simulink model "ModelForAdapt2019"  (R2019b)
settings: Solver=VariableStepAuto  StartTime=0.0  StopTime=i*dt  RelTol=1e-3
values from neighbouring files (symbols this model uses):
  t_sample_est = 0.1    [Filters.m]
undefined symbols (not defined in the file or in its folder): A, B, C, d, E, n_paramConverge, t_observer, x0
libraries: cstblocks x11
settings Model: OrderedModelArguments=off  Creator=micha  LastModifiedBy=gscul
settings DataIOCC: ExternalInput=[u, Ta, Psi]  FinalStateName=OperPoint  InitialState=OperPoint  LoadInitialState=on  SaveFinalState=on  SaveOperatingPoint=on  SaveFormat=StructureWithTime

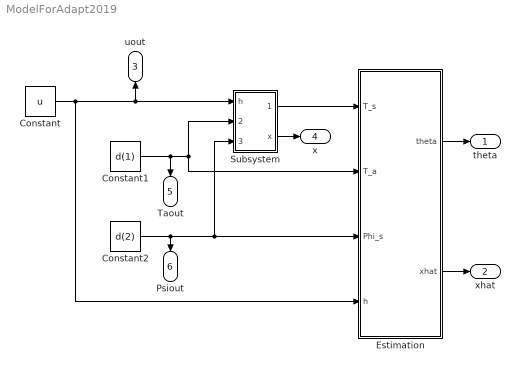
== system ModelForAdapt2019 ==
  Constant : Constant  Value=u
  Constant1 : Constant  Value=d(1)
  Constant2 : Constant  Value=d(2)
  Estimation : Subsystem
  Subsystem : Subsystem
  theta : Outport
  xhat : Outport  Port=2
  uout : Outport  Port=3
  x : Outport  Port=4
  Taout : Outport  Port=5
  Psiout : Outport  Port=6
  wires:
  Subsystem/1(T_s) -> Estimation/1(T_s)
  Estimation/1(theta) -> theta/1
  Constant2/1 -> Subsystem/3(phi_s), Estimation/3(Phi_s), Psiout/1
  Constant1/1 -> Subsystem/2(T_a), Estimation/2(T_a), Taout/1
  Estimation/2(xhat) -> xhat/1
  Constant/1 -> Estimation/4(h), uout/1, Subsystem/1(h)
  Subsystem/2(x) -> x/1

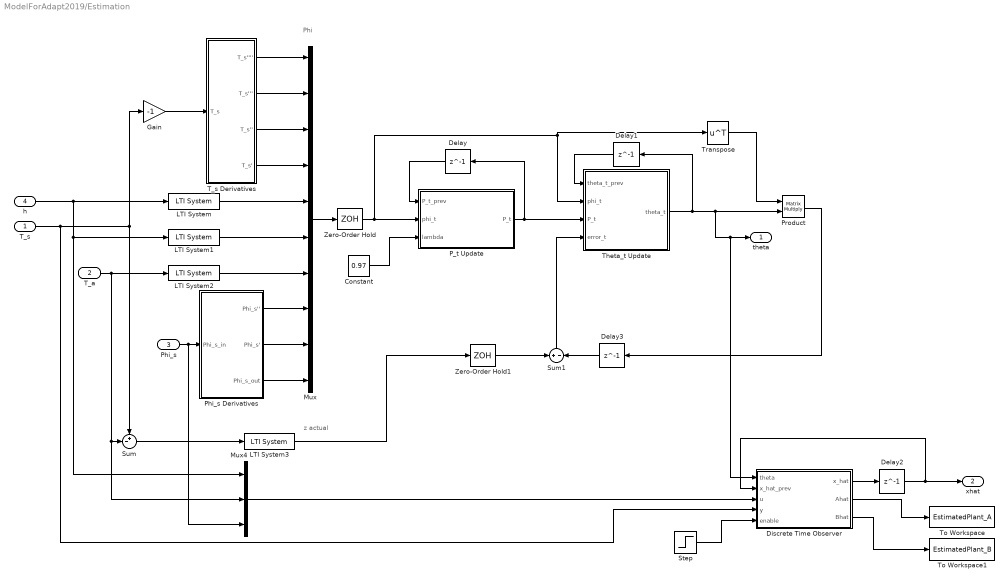
== system ModelForAdapt2019/Estimation ==
  note: Phi
  note: z actual
  T_s : Inport
  T_a : Inport  Port=2
  Phi_s : Inport  Port=3
  h : Inport  Port=4
  Constant : Constant  Value=0.97
  Delay : Delay  DelayLength=1  InitialCondition=5*eye(10)
  Delay1 : Delay  DelayLength=1  InitialCondition=0
  Delay2 : Delay  DelayLength=1  InitialCondition=[0;0;0;0];
  Delay3 : Delay  DelayLength=1  InitialCondition=0
  Discrete Time Observer : MATLAB Function  TreatAsAtomicUnit=on  SystemSampleTime=t_observer
  Gain : Gain  Gain=-1
  LTI System : cstblocks/LTI System  sys=filt_tfd_1  IC=[]
  LTI System1 : cstblocks/LTI System  sys=filt_tfd  IC=[]
  LTI System2 : cstblocks/LTI System  sys=filt_tfd_1  IC=[]
  LTI System3 : cstblocks/LTI System  sys=filt_tfd  IC=[]
  Mux : Mux  Inputs=10
  Mux4 : Mux  Inputs=3
  P_t Update : MATLAB Function  TreatAsAtomicUnit=on
  Phi_s Derivatives : Subsystem
  Product : Product  Multiplication=Matrix(*)
  Step : Step  Time=n_paramConverge
  Sum : Sum  Inputs=+-|
  Sum1 : Sum  Inputs=+|-
  T_s Derivatives : Subsystem
  Theta_t Update : MATLAB Function  TreatAsAtomicUnit=on
  To Workspace : ToWorkspace  VariableName=EstimatedPlant_A  SaveFormat=Structure  SampleTime=-1
      settings: MaxDataPoints=1
  To Workspace1 : ToWorkspace  VariableName=EstimatedPlant_B  SaveFormat=Structure  SampleTime=-1
      settings: MaxDataPoints=1
  Transpose : Math  Operator=transpose  SignedPower=off  SaturateOnIntegerOverflow=on
  Zero-Order Hold : ZeroOrderHold  SampleTime=t_sample_est
  Zero-Order Hold1 : ZeroOrderHold  SampleTime=t_sample_est
  theta : Outport
  xhat : Outport  Port=2
  wires:
  T_a/1 -> LTI System2/1, Mux4/2, Sum/2
  Gain/1 -> T_s Derivatives/1(T_s)
  Phi_s/1 -> Mux4/3, Phi_s Derivatives/1(Phi_s_in)
  h/1 -> LTI System/1, LTI System1/1, Mux4/1
  T_s Derivatives/1(T_s'''') -> Mux/1
  T_s Derivatives/2(T_s''') -> Mux/2
  T_s Derivatives/3(T_s'') -> Mux/3
  T_s Derivatives/4(T_s') -> Mux/4
  P_t Update/1(P_t) -> Delay/1, Theta_t Update/3(P_t)
  Mux/1 -> Zero-Order Hold/1
  Constant/1 -> P_t Update/3(lambda)
  Delay/1 -> P_t Update/1(P_t_prev)
  Delay1/1 -> Theta_t Update/1(theta_t_prev)
  LTI System/1 -> Mux/5
  LTI System1/1 -> Mux/6
  Sum/1 -> LTI System3/1
  LTI System3/1 -> Zero-Order Hold1/1
  Sum1/1 -> Theta_t Update/4(error_t)
  Zero-Order Hold1/1 -> Sum1/1
  Transpose/1 -> Product/1
  Zero-Order Hold/1 -> Theta_t Update/2(phi_t), Transpose/1, P_t Update/2(phi_t)
  LTI System2/1 -> Mux/7
  Phi_s Derivatives/1(Phi_s'') -> Mux/8
  Phi_s Derivatives/2(Phi_s') -> Mux/9
  Phi_s Derivatives/3(Phi_s_out) -> Mux/10
  Step/1 -> Discrete Time Observer/5(enable)
  Delay2/1 -> Discrete Time Observer/2(x_hat_prev), xhat/1
  Theta_t Update/1(theta_t) -> theta/1, Discrete Time Observer/1(theta), Product/2, Delay1/1
  Mux4/1 -> Discrete Time Observer/3(u)
  T_s/1 -> Discrete Time Observer/4(y), Gain/1, Sum/1
  Discrete Time Observer/1(x_hat) -> Delay2/1
  Delay3/1 -> Sum1/2
  Product/1 -> Delay3/1
  Discrete Time Observer/2(Ahat) -> To Workspace/1
  Discrete Time Observer/3(Bhat) -> To Workspace1/1

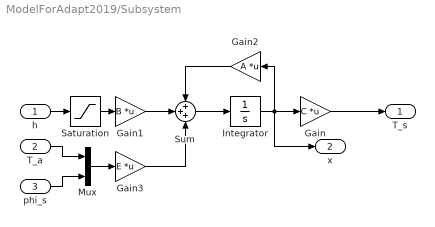
== system ModelForAdapt2019/Subsystem ==
  h : Inport
  T_a : Inport  Port=2
  phi_s : Inport  Port=3
  Gain : Gain  InitFcn=parameters  Gain=C  Multiplication=Matrix(K*u)
  Gain1 : Gain  Gain=B  Multiplication=Matrix(K*u)
  Gain2 : Gain  Gain=A  Multiplication=Matrix(K*u)
  Gain3 : Gain  Gain=E  Multiplication=Matrix(K*u)
  Integrator : Integrator  InitialCondition=x0
  Mux : Mux  Inputs=2
  Saturation : Saturate  UpperLimit=1  LowerLimit=0
  Sum : Sum  Inputs=+++
  T_s : Outport
  x : Outport  Port=2
  wires:
  Saturation/1 -> Gain1/1
  Gain/1 -> T_s/1
  Integrator/1 -> x/1, Gain2/1, Gain/1
  Gain2/1 -> Sum/1
  T_a/1 -> Mux/1
  phi_s/1 -> Mux/2
  Mux/1 -> Gain3/1
  h/1 -> Saturation/1
  Gain3/1 -> Sum/3
  Sum/1 -> Integrator/1
  Gain1/1 -> Sum/2

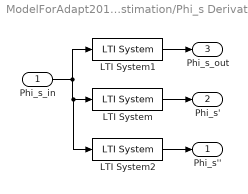
== system ModelForAdapt2019/Estimation/Phi_s Derivatives ==
  Phi_s_in : Inport
  LTI System : cstblocks/LTI System  sys=filt_tfd_1  IC=[]
  LTI System1 : cstblocks/LTI System  sys=filt_tfd  IC=[]
  LTI System2 : cstblocks/LTI System  sys=filt_tfd_2  IC=[]
  Phi_s'' : Outport
  Phi_s' : Outport  Port=2
  Phi_s_out : Outport  Port=3
  wires:
  LTI System1/1 -> Phi_s_out/1
  Phi_s_in/1 -> LTI System1/1, LTI System2/1, LTI System/1
  LTI System/1 -> Phi_s'/1
  LTI System2/1 -> Phi_s''/1

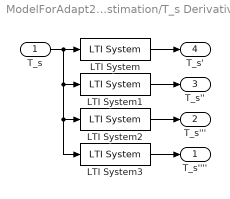
== system ModelForAdapt2019/Estimation/T_s Derivatives ==
  T_s : Inport
  LTI System : cstblocks/LTI System  sys=filt_tfd_1  IC=[]
  LTI System1 : cstblocks/LTI System  sys=filt_tfd_2  IC=[]
  LTI System2 : cstblocks/LTI System  sys=filt_tfd_3  IC=[]
  LTI System3 : cstblocks/LTI System  sys=filt_tfd_4  IC=[]
  T_s'''' : Outport
  T_s''' : Outport  Port=2
  T_s'' : Outport  Port=3
  T_s' : Outport  Port=4
  wires:
  T_s/1 -> LTI System3/1, LTI System2/1, LTI System1/1, LTI System/1
  LTI System/1 -> T_s'/1
  LTI System1/1 -> T_s''/1
  LTI System2/1 -> T_s'''/1
  LTI System3/1 -> T_s''''/1

== matlab function ModelForAdapt2019/Estimation/P_t Update ==
  data: P_t_prev input; phi_t input; P_t output; lambda input
function P_t = fcn(P_t_prev, phi_t, lambda)
% Calculate new P
  numerator   = P_t_prev*(phi_t*phi_t')*P_t_prev;
  denominator = lambda + phi_t'*P_t_prev*phi_t;

  P_t = (P_t_prev - numerator/denominator)/lambda;
end

== matlab function ModelForAdapt2019/Estimation/Theta_t Update ==
  data: theta_t_prev input; theta_t output; phi_t input; P_t input; error_t input
function theta_t = fcn(theta_t_prev, phi_t, P_t, error_t)
% Update estimation vector theta 
  delta = P_t*phi_t.*error_t;
  theta_t = theta_t_prev + delta;
end

== matlab function ModelForAdapt2019/Estimation/Discrete Time Observer ==
  data: theta input; x_hat output; x_hat_prev input; u input; y input; enable input; Ahat output; Bhat output
function [x_hat, Ahat, Bhat] = fcn(theta, x_hat_prev, u, y, enable)
  % Implement adaptive observer discretized using forward Euler
  if enable == 0
    x_hat = [0;0;0;0;];
    Ahat = zeros(4,4);
    Bhat = zeros(4,3);
  else
    Ts = 0.01; % must match sample rate of simulink block
    a_star = [22;179;638;840;]; % Cont. time eig-vals at -4, -5, -6, -7
    a4 = theta(1);
    
    % Convert plant param. estimates to _hat format
    a3_hat = theta(2)/a4;
    a2_hat = theta(3)/a4;
    a1_hat = theta(4)/a4;
    a0_hat = 1/a4;
    b1H_hat = theta(5)/a4;
    b0H_hat = theta(6)/a4;
    b1a_hat = theta(7)/a4;
    b2s_hat = theta(8)/a4;
    b1s_hat = theta(9)/a4;
    b0s_hat = theta(10)/a4;
    
    % Observer canonical form
    A_hat = [-[a3_hat;a2_hat;a1_hat;a0_hat;] ...
              [eye(3);zeros(1,3);]];
    B_hat = [0       0       0;
             0       0       b2s_hat;
             b1H_hat b1a_hat b1s_hat;
             b0H_hat a0_hat  b0s_hat;];
    
    % Forward Euler
    A_hat_d = A_hat*Ts + eye(4);
    B_hat_d = B_hat*Ts;
    
    % Error signal
    err = y - x_hat_prev(1);
    
    % Discretized adaptive observer equation
    x_hat = A_hat_d*x_hat_prev + B_hat_d*u + Ts*(a_star + A_hat(:,1)).*err;
    
    Ahat = A_hat_d;
    Bhat = B_hat_d;
  end
end
